simulink model "ACCTestBenchExample"  (R2017b)
settings: Solver=FixedStepAuto  StartTime=0.0  StopTime=34  FixedStep=0.1  RelTol=1e-3
PostLoadFcn:
  | helperACCSetUp
values from neighbouring files (symbols this model uses):
  Cf = 19000    [helperACCSetUp.m]
  Cr = 33000    [helperACCSetUp.m]
  driver_I = 0.1    [helperACCSetUp.m]
  driver_P = 0.2    [helperACCSetUp.m]
  Iz = 2875    [helperACCSetUp.m]
  lf = 1.2    [helperACCSetUp.m]
  lr = 1.6    [helperACCSetUp.m]
  m = 1575    [helperACCSetUp.m]
  R = 760    [helperACCSetUp.m]
  tau = 0.5    [helperACCSetUp.m]
  Ts = 0.1    [helperACCSetUp.m]
  v0_ego = 20.6    [helperACCSetUp.m]
  x0_ego = 0    [helperACCSetUp.m]
  y0_ego = -757.8    [helperACCSetUp.m]
  yawerr_gain = 2    [helperACCSetUp.m]
undefined symbols (not defined in the file or in its folder): driving, intmax
libraries: simulink x2, drivinglib x2, drivingmisc x1
settings Model: SnapshotInterval=5  Creator=The MathWorks, Inc.  LastModifiedBy=The MathWorks, Inc.
settings OptimizationCC: DefaultParameterBehavior=Inlined  InlineInvariantSignals=on  PassReuseOutputArgsAs=Individual arguments  ZeroExternalMemoryAtStartup=off  OptimizeBlockOrder=speed
settings DebuggingCC: ParameterTunabilityLossMsg=error
settings HardwareCC: ProdLongLongMode=on
settings ModelReferenceCC: ModelReferenceNumInstancesAllowed=Single  PropagateVarSize=Only when enabling
settings RTWCC: SystemTargetFile=ert.tlc  TemplateMakefile=ert_default_tmf  GenerateReport=on  BuildConfiguration=Faster Runs  IncludeHyperlinkInReport=on  LaunchReport=on  GenerateTraceInfo=on  GenerateTraceReport=on  GenerateTraceReportSl=on  GenerateTraceReportSf=on  GenerateTraceReportEml=on  GenerateCodeMetricsReport=on
settings CodeAppCC: ForceParamTrailComments=on  IgnoreCustomStorageClasses=off  OperatorAnnotations=on  SimulinkDataObjDesc=on  SFDataObjDesc=on  CustomSymbolStrFcn=$N$M$F  InsertBlockDesc=on
settings ERTTargetCC: TargetLangStandard=C99 (ISO)  GenerateSampleERTMain=on  CombineSignalStateStructs=on  SuppressErrorStatus=on  InlinedParameterPlacement=NonHierarchical  RootIOFormat=Structure reference  RTWCAPISignals=on  ERTCustomFileTemplate=example_file_process.tlc

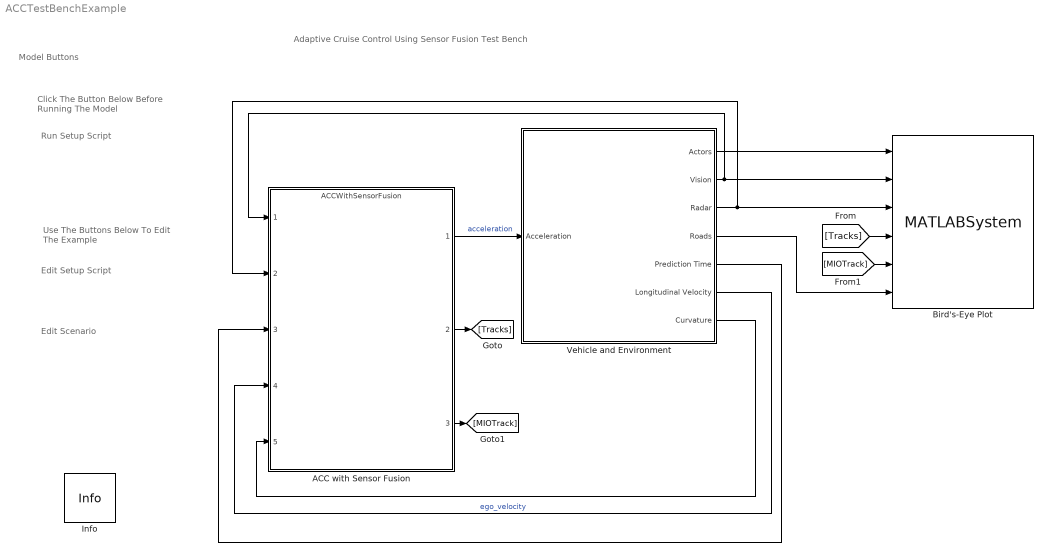
== system ACCTestBenchExample ==
  note: Click The Button Below Before Running The Model
  note: Model Buttons
  note: Adaptive Cruise Control Using Sensor Fusion Test Bench
  note: Edit Setup Script
  note: Edit Scenario
  note: Run Setup Script
  note: Use The Buttons Below To Edit The Example
  ACC with Sensor Fusion : ModelReference  ModelNameDialog=ACCWithSensorFusion.slx  SimulationMode=Normal  CodeInterface=Top model  ModelReferenceVersion=1.455
  Bird's-Eye Plot : MATLABSystem  System=helperBirdsEyePlot  XLim=[ -10, 200 ]  YLim=[ -50, 50 ]  HasActors=on  HasVision=on  HasRadar=on  HasTracks=on  TrackPositionSelector=posSelector  TrackVelocitySelector=velSelector  HasMIO=on  HasRoads=on
      settings: ModelCloseFcn=helperCloseAll(gcb)
      mask Type: helperBirdsEyePlot
      mask Display:
      | disp(['Bird''s-Eye' char(10) 'Plot']);
      | port_label('input',1,'Actors');
      | port_label('input',2,'Vision');
      | port_label('input',3,'Radar');
      | port_label('input',4,'Tracks');
      | port_label('input',5,'MIO');
      | port_label('input',6,'Roads');
  Info : drivingmisc/Info  SystemSampleTime=-1
      settings: AttributesFormatString=%<Name>  SourceProductName=Computer Vision System Toolbox  SourceProductBaseCode=VP
  Vehicle and Environment : Subsystem
  wires:
  [Tracks] -> Bird's-Eye Plot/4
  Vehicle and Environment/1(Actors) -> Bird's-Eye Plot/1
  Vehicle and Environment/2(Vision) -> ACC with Sensor Fusion/1, Bird's-Eye Plot/2
  Vehicle and Environment/3(Radar) -> ACC with Sensor Fusion/2, Bird's-Eye Plot/3
  [MIOTrack] -> Bird's-Eye Plot/5
  Vehicle and Environment/4(Roads) -> Bird's-Eye Plot/6
  Vehicle and Environment/5(Prediction Time) -> ACC with Sensor Fusion/3
  Vehicle and Environment/6(Longitudinal Velocity) -> ACC with Sensor Fusion/4  "ego_velocity"
  Vehicle and Environment/7(Curvature) -> ACC with Sensor Fusion/5
  ACC with Sensor Fusion/1 -> Vehicle and Environment/1(Acceleration)  "acceleration"
  ACC with Sensor Fusion/2 -> [Tracks]
  ACC with Sensor Fusion/3 -> [MIOTrack]

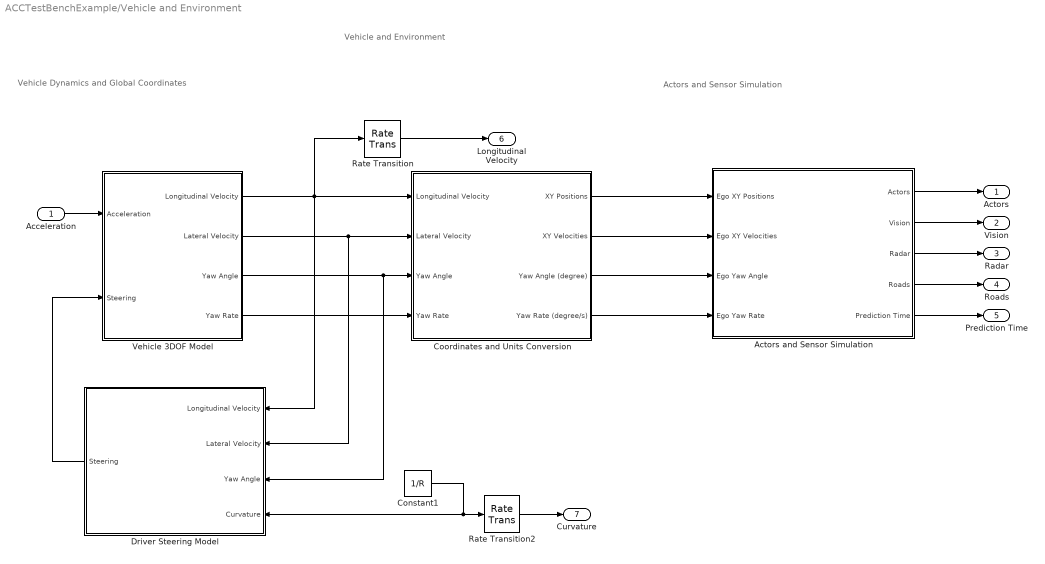
== system ACCTestBenchExample/Vehicle and Environment ==
  note: Actors and Sensor Simulation
  note: Vehicle Dynamics and Global Coordinates
  note: Vehicle and Environment
  Acceleration : Inport  OutDataTypeStr=double  PortDimensions=1
  "  Vehicle 3DOF Model " : Subsystem
  Actors and Sensor Simulation : Subsystem
  Constant1 : Constant  Value=1/R
  Coordinates and Units Conversion : Subsystem
  Driver Steering Model : Subsystem
  Rate Transition : RateTransition  OutPortSampleTime=Ts
  Rate Transition2 : RateTransition  OutPortSampleTime=Ts
  Actors : Outport
  Vision : Outport  Port=2
  Radar : Outport  Port=3
  Roads : Outport  Port=4
  Prediction Time : Outport  Port=5
  Longitudinal Velocity : Outport  Port=6
  Curvature : Outport  Port=7
  wires:
  Actors and Sensor Simulation/2(Vision) -> Vision/1
  Actors and Sensor Simulation/3(Radar) -> Radar/1
  Actors and Sensor Simulation/5(Prediction Time) -> Prediction Time/1
  Actors and Sensor Simulation/4(Roads) -> Roads/1
  Actors and Sensor Simulation/1(Actors) -> Actors/1
  Rate Transition2/1 -> Curvature/1
  "  Vehicle 3DOF Model "/1(Longitudinal Velocity) -> Driver Steering Model/1(Longitudinal Velocity), Rate Transition/1, Coordinates and Units Conversion/1(Longitudinal Velocity)
  Rate Transition/1 -> Longitudinal Velocity/1
  Coordinates and Units Conversion/4(Yaw Rate (degree/s)) -> Actors and Sensor Simulation/4(Ego Yaw Rate)
  "  Vehicle 3DOF Model "/3(Yaw Angle) -> Driver Steering Model/3(Yaw Angle), Coordinates and Units Conversion/3(Yaw Angle)
  Coordinates and Units Conversion/1(XY Positions) -> Actors and Sensor Simulation/1(Ego XY Positions)
  Coordinates and Units Conversion/3(Yaw Angle (degree)) -> Actors and Sensor Simulation/3(Ego Yaw Angle)
  "  Vehicle 3DOF Model "/4(Yaw Rate) -> Coordinates and Units Conversion/4(Yaw Rate)
  "  Vehicle 3DOF Model "/2(Lateral Velocity) -> Driver Steering Model/2(Lateral Velocity), Coordinates and Units Conversion/2(Lateral Velocity)
  Coordinates and Units Conversion/2(XY Velocities) -> Actors and Sensor Simulation/2(Ego XY Velocities)
  Acceleration/1 -> "  Vehicle 3DOF Model "/1(Acceleration)
  Constant1/1 -> Driver Steering Model/4(Curvature), Rate Transition2/1
  Driver Steering Model/1(Steering) -> "  Vehicle 3DOF Model "/2(Steering)

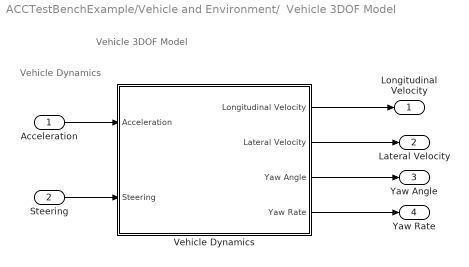
== system ACCTestBenchExample/Vehicle and Environment/  Vehicle 3DOF Model  ==
  note: Vehicle Dynamics
  note: Vehicle 3DOF Model
  Acceleration : Inport
  Steering : Inport  Port=2
  Vehicle Dynamics : Subsystem
  Longitudinal Velocity : Outport
  Lateral Velocity : Outport  Port=2
  Yaw Angle : Outport  Port=3
  Yaw Rate : Outport  Port=4
  wires:
  Steering/1 -> Vehicle Dynamics/2(Steering)
  Acceleration/1 -> Vehicle Dynamics/1(Acceleration)
  Vehicle Dynamics/1(Longitudinal Velocity) -> Longitudinal Velocity/1
  Vehicle Dynamics/2(Lateral Velocity) -> Lateral Velocity/1
  Vehicle Dynamics/3(Yaw Angle) -> Yaw Angle/1
  Vehicle Dynamics/4(Yaw Rate) -> Yaw Rate/1

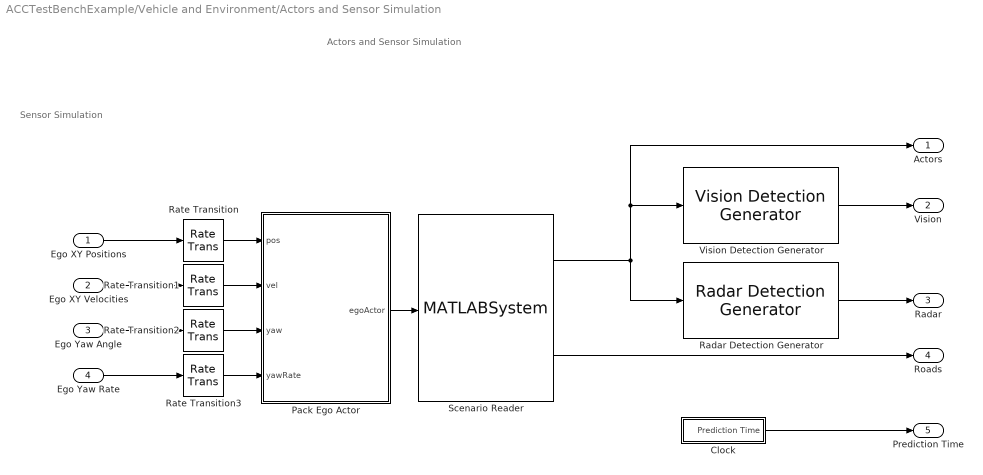
== system ACCTestBenchExample/Vehicle and Environment/Actors and Sensor Simulation ==
  note: Sensor Simulation
  note: Actors and Sensor Simulation
  Ego XY Positions : Inport
  Ego XY Velocities : Inport  Port=2
  Ego Yaw Angle : Inport  Port=3
  Ego Yaw Rate : Inport  Port=4
  Clock : Subsystem
  Pack Ego Actor : MATLAB Function  TreatAsAtomicUnit=on
  Radar Detection Generator : drivinglib/Radar Detection Generator  SensorIndex=2  UpdateInterval=0.1  SensorLocation=[ 3.7, 0 ]  Height=0.2  Yaw=0  Pitch=0  Roll=0  BusNameSource=Property  BusName=BusRadar  MaxNumDetectionsSource=Property  MaxNumDetections=50  DetectionCoordinates=Ego Cartesian  SimulateUsing=Interpreted execution  AzimuthResolution=4  ElevationResolution=10  RangeResolution=2.5  RangeRateResolution=0.5  AzimuthBiasFraction=0.1  ElevationBiasFraction=0.1  RangeBiasFraction=0.05  RangeRateBiasFraction=0.05  FieldOfView=[ 20, 5 ]  MaxRange=174  RangeRateLimits=[ -100, 100 ]  DetectionProbability=0.9  FalseAlarmRate=1e-6  ReferenceRange=100  ReferenceRCS=0  HasElevation=off  HasRangeRate=on  HasNoise=on  HasFalseAlarms=on  InitialSeedSource=Repeatable  InitialSeed=0  UsedSeed=driving.internal.SimulinkUtilities.seedManager(gcb)  ActorProfilesSource=Parameters  ActorProfilesParameters=driving.internal.ActorProfilesRadarParameters  ActorProfilesExpression=struct( 'ClassID', 0, 'Length', 4.7, 'Width', 1.8, 'Height', 1.4, 'OriginOffset', [ -1.35, 0, 0 ], 'RCSPattern', [ 10, 10; 10, 10 ], 'RCSAzimuthAngles', [ -180, 180 ], 'RCSElevationAngles', [ -90, 90 ] )
      settings: SourceProductName=Automated Driving System Toolbox
  Rate Transition{,1..3} (4 alike) : RateTransition  OutPortSampleTime=Ts
  Scenario Reader : MATLABSystem  System=helperScenarioReader  ScenarioFileName=ACCscenario  EgoActorSource=Input port  EgoActorID=1  RoadBoundaries=on  BusNameSource=Property  BusName=BusActors  SimulateUsing=Interpreted execution
      mask Type: helperScenarioReader
      mask Display:
      | disp(['Scenario' char(10) 'Reader']);
      | port_label('input',1,'Ego Actor');
      | port_label('output',1,'Actors');
      | port_label('output',2,'Roads');
  Vision Detection Generator : drivinglib/Vision Detection Generator  SensorIndex=1  UpdateInterval=0.1  SensorLocation=[ 2.1, 0 ]  Height=1.1  Yaw=0  Pitch=1  Roll=0  BusNameSource=Property  BusName=BusVision  MaxNumDetectionsSource=Property  MaxNumDetections=20  DetectionCoordinates=Ego Cartesian  SimulateUsing=Interpreted execution  BoundingBoxAccuracy=5  ProcessNoiseIntensity=5  HasNoise=on  MaxRange=150  MaxSpeed=50  MaxAllowedOcclusion=0.5  MinObjectImageSize=[ 15, 15 ]  DetectionProbability=0.9  FalsePositivesPerImage=0.1  InitialSeedSource=Repeatable  InitialSeed=0  UsedSeed=driving.internal.SimulinkUtilities.seedManager(gcb)  ActorProfilesSource=Parameters  ActorProfilesParameters=driving.internal.ActorProfilesParameters  ActorProfilesExpression=struct( 'ClassID', 0, 'Length', 4.7, 'Width', 1.8, 'Height', 1.4, 'OriginOffset', [ -1.35, 0, 0 ] )  Intrinsics=driving.internal.cameraIntrinsics
      settings: SourceProductName=Automated Driving System Toolbox
  Actors : Outport
  Vision : Outport  Port=2
  Radar : Outport  Port=3
  Roads : Outport  Port=4
  Prediction Time : Outport  Port=5
  wires:
  Rate Transition3/1 -> Pack Ego Actor/4(yawRate)
  Scenario Reader/2 -> Roads/1
  Rate Transition1/1 -> Pack Ego Actor/2(vel)
  Rate Transition2/1 -> Pack Ego Actor/3(yaw)
  Ego XY Positions/1 -> Rate Transition/1
  Ego Yaw Rate/1 -> Rate Transition3/1
  Scenario Reader/1 -> Radar Detection Generator/1, Vision Detection Generator/1, Actors/1
  Rate Transition/1 -> Pack Ego Actor/1(pos)
  Ego Yaw Angle/1 -> Rate Transition2/1
  Vision Detection Generator/1 -> Vision/1
  Clock/1(Prediction Time) -> Prediction Time/1
  Ego XY Velocities/1 -> Rate Transition1/1
  Pack Ego Actor/1(egoActor) -> Scenario Reader/1
  Radar Detection Generator/1 -> Radar/1

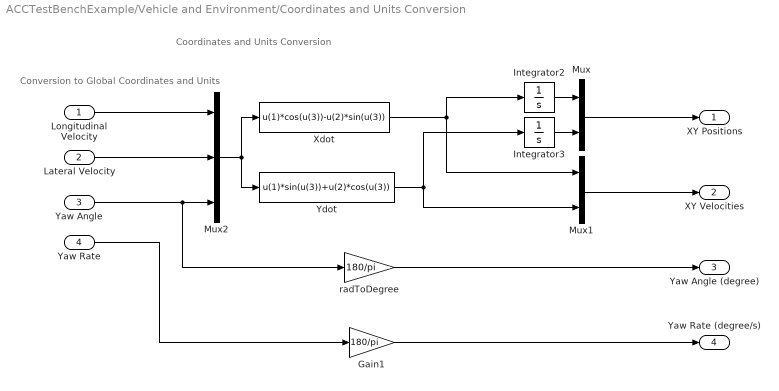
== system ACCTestBenchExample/Vehicle and Environment/Coordinates and Units Conversion ==
  note: Conversion to Global Coordinates and Units
  note: Coordinates and Units Conversion
  Longitudinal Velocity : Inport
  Lateral Velocity : Inport  Port=2
  Yaw Angle : Inport  Port=3
  Yaw Rate : Inport  Port=4
  Gain1 : Gain  Gain=180/pi
  Integrator2 : Integrator  InitialCondition=x0_ego
  Integrator3 : Integrator  InitialCondition=y0_ego
  Mux : Mux  Inputs=2
  Mux1 : Mux  Inputs=2
  Mux2 : Mux  Inputs=3
  Xdot : Fcn  Expr=u(1)*cos(u(3))-u(2)*sin(u(3))
  Ydot : Fcn  Expr=u(1)*sin(u(3))+u(2)*cos(u(3))
  "radToDegree " : Gain  Gain=180/pi
  XY Positions : Outport
  XY Velocities : Outport  Port=2
  Yaw Angle (degree) : Outport  Port=3
  Yaw Rate (degree/s) : Outport  Port=4
  wires:
  "radToDegree "/1 -> Yaw Angle (degree)/1
  Integrator2/1 -> Mux/1
  Mux/1 -> XY Positions/1
  Ydot/1 -> Mux1/2, Integrator3/1
  Gain1/1 -> Yaw Rate (degree/s)/1
  Yaw Rate/1 -> Gain1/1
  Integrator3/1 -> Mux/2
  Xdot/1 -> Integrator2/1, Mux1/1
  Mux1/1 -> XY Velocities/1
  Lateral Velocity/1 -> Mux2/2
  Mux2/1 -> Ydot/1, Xdot/1
  Longitudinal Velocity/1 -> Mux2/1
  Yaw Angle/1 -> "radToDegree "/1, Mux2/3

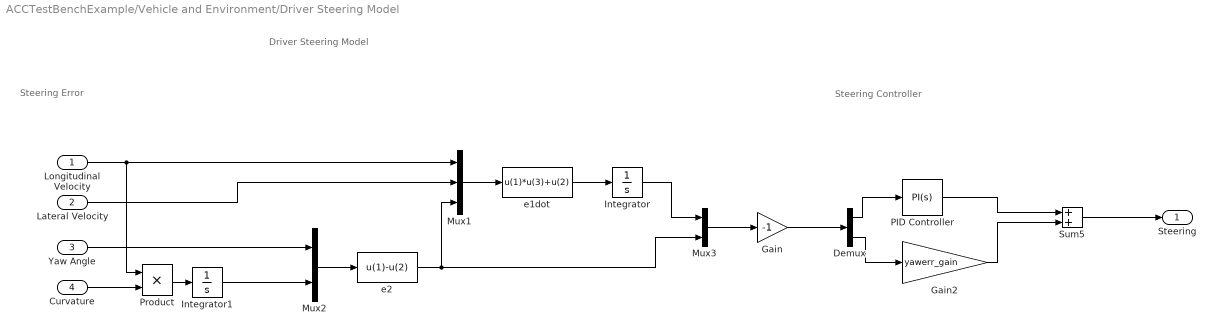
== system ACCTestBenchExample/Vehicle and Environment/Driver Steering Model ==
  note: Steering Controller
  note: Steering Error
  note: Driver Steering Model
  Longitudinal Velocity : Inport
  Lateral Velocity : Inport  Port=2
  Yaw Angle : Inport  Port=3
  Curvature : Inport  Port=4
  Demux : Demux  Outputs=2
  Gain : Gain  Gain=-1
  Gain2 : Gain  Gain=yawerr_gain
  Integrator : Integrator
  Integrator1 : Integrator
  Mux1 : Mux  Inputs=3
  Mux2 : Mux  Inputs=2
  Mux3 : Mux  Inputs=2
  PID Controller : simulink/Continuous/PID Controller  Controller=PI  TimeDomain=Continuous-time  SampleTime=-1  IntegratorMethod=Forward Euler  FilterMethod=Forward Euler  Form=Parallel  UseFilter=on  ControllerParametersSource=internal  P=driver_P  I=driver_I  D=0  N=100  InitialConditionSource=internal  InitialConditionForIntegrator=0  InitialConditionForFilter=0  ExternalReset=none  LimitOutput=off  UpperSaturationLimit=inf  LowerSaturationLimit=-inf  LinearizeAsGain=on  AntiWindupMode=none  Kb=1  TrackingMode=off  Kt=1  PParamMin=[]  PParamMax=[]  IParamMin=[]  IParamMax=[]  DParamMin=[]  DParamMax=[]  NParamMin=[]  NParamMax=[]  KbParamMin=[]  KbParamMax=[]  KtParamMin=[]  KtParamMax=[]  POutMin=[]  POutMax=[]  IOutMin=[]  IOutMax=[]  DOutMin=[]  DOutMax=[]  NOutMin=[]  NOutMax=[]  KbOutMin=[]  KbOutMax=[]  KtOutMin=[]  KtOutMax=[]  IntegratorOutMin=[]  IntegratorOutMax=[]  FilterOutMin=[]  FilterOutMax=[]  SumOutMin=[]  SumOutMax=[]  SumI1OutMin=[]  SumI1OutMax=[]  SumI2OutMin=[]  SumI2OutMax=[]  SumI3OutMin=[]  SumI3OutMax=[]  SumDOutMin=[]  SumDOutMax=[]  SaturationOutMin=[]  SaturationOutMax=[]  IntegratorContinuousStateAttributes=''  IntegratorStateMustResolveToSignalObject=off  IntegratorRTWStateStorageClass=Auto  FilterContinuousStateAttributes=''  FilterStateMustResolveToSignalObject=off  FilterRTWStateStorageClass=Auto  DifferentiatorICPrevScaledInput=0  DifferentiatorOutMin=[]  DifferentiatorOutMax=[]  InitialConditionSetting=State (most efficient)  FilterDiffOutCoefMin=[]  FilterDiffOutCoefMax=[]  SumDenOutMin=[]  SumDenOutMax=[]  SumNumOutMin=[]  SumNumOutMax=[]  ReciprocalOutMin=[]  ReciprocalOutMax=[]  DivideOutMin=[]  DivideOutMax=[]  TunerSelectOption=Transfer Function Based (PID Tuner App)
  Product : Product
  Sum5 : Sum
  e1dot : Fcn  Expr=u(1)*u(3)+u(2)
  e2 : Fcn  Expr=u(1)-u(2)
  Steering : Outport
  wires:
  e1dot/1 -> Integrator/1
  Mux2/1 -> e2/1
  e2/1 -> Mux1/3, Mux3/2
  Mux3/1 -> Gain/1
  Lateral Velocity/1 -> Mux1/2
  Yaw Angle/1 -> Mux2/1
  Mux1/1 -> e1dot/1
  Integrator/1 -> Mux3/1
  Product/1 -> Integrator1/1
  Integrator1/1 -> Mux2/2
  Curvature/1 -> Product/2
  Longitudinal Velocity/1 -> Product/1, Mux1/1
  Gain2/1 -> Sum5/2
  PID Controller/1 -> Sum5/1
  Demux/2 -> Gain2/1
  Sum5/1 -> Steering/1
  Demux/1 -> PID Controller/1
  Gain/1 -> Demux/1

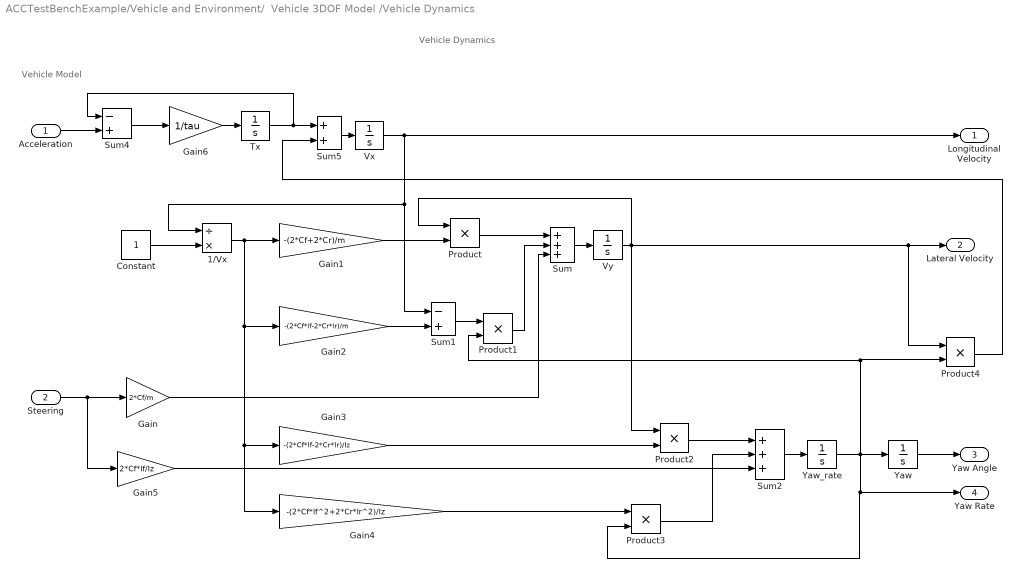
== system ACCTestBenchExample/Vehicle and Environment/  Vehicle 3DOF Model /Vehicle Dynamics ==
  note: Vehicle Model
  note: Vehicle Dynamics
  Acceleration : Inport
  Steering : Inport  Port=2
  1/Vx : Product  Inputs=/*
  Constant : Constant
  Gain : Gain  Gain=2*Cf/m
  Gain1 : Gain  Gain=-(2*Cf+2*Cr)/m
  Gain2 : Gain  Gain=-(2*Cf*lf-2*Cr*lr)/m
  Gain3 : Gain  Gain=-(2*Cf*lf-2*Cr*lr)/Iz
  Gain4 : Gain  Gain=-(2*Cf*lf^2+2*Cr*lr^2)/Iz
  Gain5 : Gain  Gain=2*Cf*lf/Iz
  Gain6 : Gain  Gain=1/tau
  Product{,1..4} (5 alike) : Product
  Sum : Sum  Inputs=+++
  Sum1 : Sum  Inputs=-+
  Sum2 : Sum  Inputs=+++
  Sum4 : Sum  Inputs=-+
  Sum5 : Sum
  Tx : Integrator
  Vx : Integrator  InitialCondition=v0_ego
  Vy : Integrator
  Yaw : Integrator
  "Yaw_rate " : Integrator
  Longitudinal Velocity : Outport
  Lateral Velocity : Outport  Port=2
  Yaw Angle : Outport  Port=3
  Yaw Rate : Outport  Port=4
  wires:
  Gain6/1 -> Tx/1
  Sum2/1 -> "Yaw_rate "/1
  Sum5/1 -> Vx/1
  Gain2/1 -> Sum1/2
  Gain4/1 -> Product3/1
  Constant/1 -> 1/Vx/2
  Gain3/1 -> Product2/2
  1/Vx/1 -> Gain4/1, Gain3/1, Gain2/1, Gain1/1
  Product2/1 -> Sum2/1
  Sum4/1 -> Gain6/1
  Acceleration/1 -> Sum4/2
  Tx/1 -> Sum5/1, Sum4/1
  Product3/1 -> Sum2/2
  Gain5/1 -> Sum2/3
  Product4/1 -> Sum5/2
  Sum1/1 -> Product1/1
  "Yaw_rate "/1 -> Yaw Rate/1, Product3/2, Product4/2, Product1/2, Yaw/1
  Gain/1 -> Sum/3
  Yaw/1 -> Yaw Angle/1
  Steering/1 -> Gain/1, Gain5/1
  Gain1/1 -> Product/2
  Product/1 -> Sum/1
  Vy/1 -> Product/1, Lateral Velocity/1, Product4/1, Product2/1
  Sum/1 -> Vy/1
  Vx/1 -> Longitudinal Velocity/1, 1/Vx/1, Sum1/1
  Product1/1 -> Sum/2

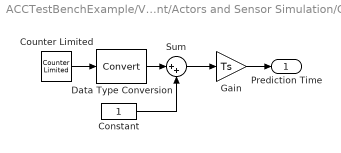
== system ACCTestBenchExample/Vehicle and Environment/Actors and Sensor Simulation/Clock ==
  Constant : Constant
  Counter Limited : simulink/Sources/Counter Limited  uplimit=intmax  tsamp=Ts
  Data Type Conversion : DataTypeConversion
  Gain : Gain  Gain=Ts
  Sum : Sum  Inputs=|++
  Prediction Time : Outport
  wires:
  Gain/1 -> Prediction Time/1
  Sum/1 -> Gain/1
  Constant/1 -> Sum/2
  Data Type Conversion/1 -> Sum/1
  Counter Limited/1 -> Data Type Conversion/1

== matlab function ACCTestBenchExample/Vehicle and Environment/Actors and Sensor Simulation/Pack Ego Actor ==
  data: pos input; egoActor output Bus: BusActorsActors size=1; vel input; yaw input; yawRate input
function egoActor = packEgo(pos,vel,yaw,yawRate)
% Pack ego information into a single ego actor bus
%
% Imoprtant note:
% Output is a bus of type BusActorsActors. This is the same bus used by the
% helperScenarioReader to output an individual actor. If you change the
% output bus name of helperScenarioReader, change the output bus name here
% as well by clicking on 'Edit Data' in the menu above.

egoActor = struct(...
    'ActorID',1,...
    'Position', [pos(1) pos(2) 0], ...
    'Velocity', [vel(1) vel(2) 0], ...
    'Roll', 0, ...
    'Pitch', 0, ...
    'Yaw', yaw, ...
    'AngularVelocity', [0 0 yawRate]);
